simulink model "six_plus_six_AcmsteeringV09_main_2lfrf"  (R2014a)
settings: Solver=FixedStepDiscrete  StartTime=0.0  StopTime=10.0  FixedStep=0.0005  RelTol=1e-3
InitFcn:
  | Veh_Par_wxt
undefined symbols (not defined in the file or in its folder): acc_spdctl, ag_thr, B, bra_em, bra_pre_gz2, bra_pre_gz34, bra_pre_yd, brakepre_dem_data, brakeTrq_dem_data, bratrq_max, ecucoder_acal, eff_tran, ESP_switch, G, guzhang_lf, guzhang_lm, guzhang_lr, guzhang_rf, guzhang_rm, guzhang_rr, kd1, kd2, ki1, ki2, kp1, kp2, L, myFIS, premax, Radius, RC_switch, s_opt_yi, s_opt_zhuan, s_opt_zhuan_add, s_opt_zhuan_table, spd_map_mot, spd_spdctl, speed_thr_park, TCS_switch, tras_ratio, trq_map_mot, trqmax_yd, trqmax_zx, trqmaxneg, v_gain, v_table, v_thr_park, zhidong_bianmazhi, zhidong_down, zhidong_up, zhidong_youmen, zhuanxiang_bianmazhi, zhuanxiang_down, zhuanxiang_up, zhuanxiang_youmen
libraries: simulink x980, ec5744lib x59, fuzblock x2
(part 1 of 25)
settings Model: Creator=pc  LastModifiedBy=ZJK
settings OptimizationCC: InlineParams=on  InlineInvariantSignals=on  ExpressionFolding=off  RollThreshold=9  StateBitsets=on  DataBitsets=on  UseTempVars=on  ZeroExternalMemoryAtStartup=off  ZeroInternalMemoryAtStartup=off  EfficientFloat2IntCast=on  OptimizeModelRefInitCode=on  LifeSpan=1
settings DebuggingCC: InheritedTsInSrcMsg=none  MultiTaskDSMMsg=none
settings HardwareCC: ProdLargestAtomicInteger=Long  ProdLargestAtomicFloat=Double  ProdIntDivRoundTo=Zero  ProdEndianess=BigEndian  ProdHWDeviceType=Freescale MPC5500
settings RTWCC: SystemTargetFile=ec5744.tlc  MakeCommand=make_rtw optimized_fixed_point=1  GenerateMakefile=off  TemplateMakefile=ec5744_lcc.tmf  PostCodeGenCommand=ec5744_pst_s2(buildInfo)  Description=Target for EC5744  GenerateReport=on  ProcessScript=ec5744_make_rtw_hook  IncludeHyperlinkInReport=on  LaunchReport=on
settings CodeAppCC: IgnoreCustomStorageClasses=off
settings STFCustomTargetCC: ModelReferenceCompliant=off  ConcurrentExecutionCompliant=off  IncludeMdlTerminateFcn=off  GeneratePreprocessorConditionals=Use local settings  CombineOutputUpdateFcns=on  SuppressErrorStatus=on  ERTCustomFileBanners=on  SupportContinuousTime=off  SupportNonInlinedSFcns=off  MATLABClassNameForMDSCustomization=Simulink.SoftwareTarget.ERTCustomization  GRTInterface=off  SystemTargetFile=ec5744.tlc
settings ERTTargetCC: GenerateSampleERTMain=off  ModelReferenceCompliant=off  IncludeMdlTerminateFcn=off  SuppressErrorStatus=on  GenerateASAP2=on  ERTSrcFileBannerTemplate=ec5744_code_template.cgt  ERTHdrFileBannerTemplate=ec5744_code_template.cgt  ERTDataSrcFileTemplate=ec5744_code_template.cgt  ERTDataHdrFileTemplate=ec5744_code_template.cgt  ERTCustomFileTemplate=ec5744_file_process.tlc

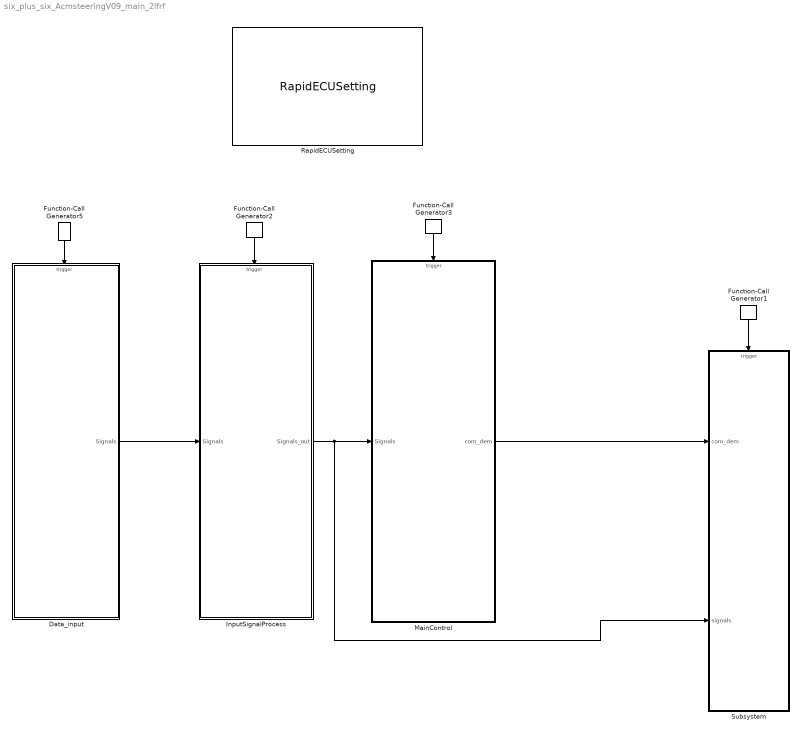
== system six_plus_six_AcmsteeringV09_main_2lfrf ==
  Data_input : Subsystem
  Function-Call Generator{1..3,5} (4 alike) : simulink/Ports & Subsystems/Function-Call Generator  sample_time=0.05  numberOfIterations=1
  InputSignalProcess : Subsystem  TreatAsAtomicUnit=on
  MainControl : Subsystem
  RapidECUSetting : ec5744lib/RapidECU_U3/RapidECUSetting
      link override CAN: apdf=4  bpdf=4  cpdf=4  acmt=Extended(29-bit ID)
      link override LIN: abrt=19200
  Subsystem : Subsystem
  wires:
  Function-Call Generator5/1 -> Data_input/Trigger
  Function-Call Generator1/1 -> Subsystem/Trigger
  Data_input/1(Signals) -> InputSignalProcess/1(Signals)
  Function-Call Generator2/1 -> InputSignalProcess/Trigger
  Function-Call Generator3/1 -> MainControl/Trigger
  InputSignalProcess/1(Signals_out) -> Subsystem/2("signals "), MainControl/1(Signals)
  MainControl/1(com_dem) -> Subsystem/1(com_dem)

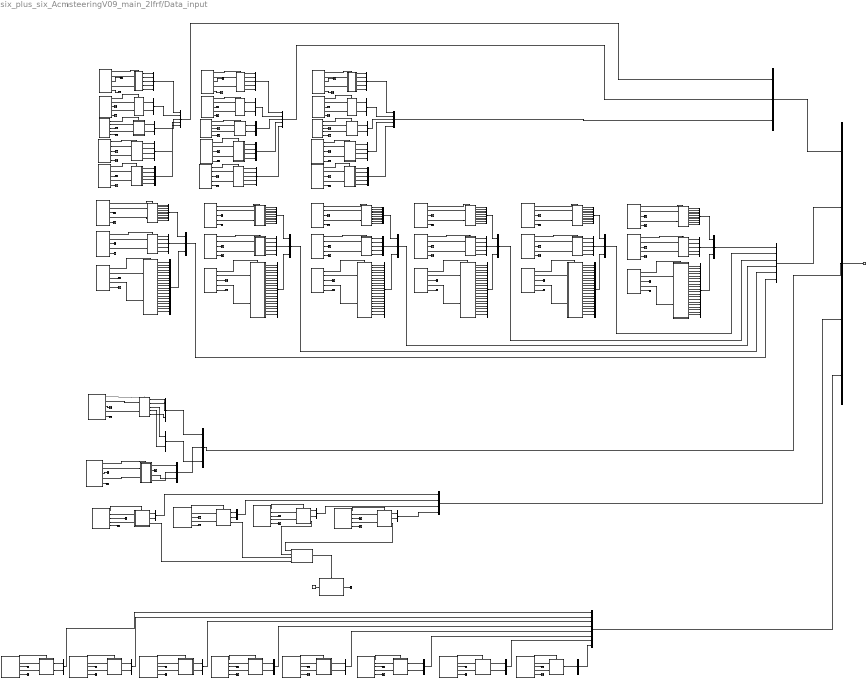
== system six_plus_six_AcmsteeringV09_main_2lfrf/Data_input ==
  note: 驱动电机1
  note: 电池管理系统主机1
  note: 电机报警信息
  note: 电机电气参数
  note: 电机状态信息
  note: 电池管理系统主机2
  note: 电池管理系统主机3
  note: 驱动电机2
  note: 电机报警信息
  note: 电机电气参数
  note: 电机状态信息
  note: 驱动电机3
  note: 电机报警信息
  note: 电机电气参数
  note: 电机状态信息
  note: 驱动电机4
  note: 电机报警信息
  note: 电机电气参数
  note: 电机状态信息
  note: 驱动电机5
  note: 电机报警信息
  note: 电机电气参数
  note: 电机状态信息
  note: 驱动电机6
  note: 电机报警信息
  note: 电机电气参数
  note: 电机状态信息
  note: 遥控器1
  note: SH/SE/ SD/SA/ 生命信号
  note: 遥控器2
  note: 左右摇杆
  note: motec转向电机1反馈报文
  note: motec转向电机2反馈报文
  note: motec转向电机3反馈报文
  note: motec制动电机反馈报文
  note: 进入OP模式，预设2s
  note: 组合惯导反馈报文1
  note: 组合惯导反馈报文2
  note: 组合惯导反馈报文3
  note: 组合惯导反馈报文4
  note: 组合惯导反馈报文5
  note: 组合惯导反馈报文6
  note: 组合惯导反馈报文7
  note: 组合惯导反馈报文8
  function : TriggerPort  TriggerType=function-call
  1 : Subsystem
  10 : Subsystem
  11 : Subsystem
  181 : Subsystem
  2 : Subsystem
  3 : Subsystem
  4 : Subsystem
  5 : Subsystem
  6 : Subsystem
  7 : Subsystem
  8 : Subsystem
  9 : Subsystem
  BMS1 : Subsystem
  BMS1-2 : Subsystem
  BMS1_1 : Subsystem
  BMS2 : Subsystem
  BMS2_1 : Subsystem
  BMS2_2 : Subsystem
  BMS3 : Subsystem
  BMS3_1 : Subsystem
  BMS3_2 : Subsystem
  BMS4 : Subsystem
  BMS4_1 : Subsystem
  BMS4_2 : Subsystem
  BMS5 : Subsystem
  BMS5_1 : Subsystem
  BMS5_2 : Subsystem
  Bus Creator{,22,25,28,31,34} (6 alike) : BusCreator  Inputs=10
  Bus Creator{1,3,7..9,13..15,19..20,23,26,29,32,35,44} (16 alike) : BusCreator  Inputs=5
  Bus Creator{4..5,10..11,16..17,47,49..52,57..63} (18 alike) : BusCreator  Inputs=2
  Bus Creator{6,12,18,53} (4 alike) : BusCreator
  Bus Creator{2,24,27,30,33,36} (6 alike) : BusCreator  Inputs=20
  Bus Creator{21,37..42,45..46,48} (10 alike) : BusCreator  Inputs=3
  Bus Creator43 : BusCreator  Inputs=6
  Bus Creator64 : BusCreator  Inputs=8
  Bus Creator65 : BusCreator  Inputs=1
  CANReceive : ec5744lib/RapidECU_U3/04CANCommunication/CANReceive  canmodule=0  canbuffer=23  canmessageid=hex2dec('CFA00EF')  canmessagetype=Extended(29-bit ID)  datalength=8  sampletime=-1
  CANReceive1 : ec5744lib/RapidECU_U3/04CANCommunication/CANReceive  canmodule=0  canbuffer=24  canmessageid=hex2dec('CFA01EF')  canmessagetype=Extended(29-bit ID)  datalength=8  sampletime=-1
  CANReceive10 : ec5744lib/RapidECU_U3/04CANCommunication/CANReceive  canmodule=1  canbuffer=7  canmessageid=hex2dec('42')  canmessagetype=Standard(11-bit ID)  datalength=8  sampletime=-1
  CANReceive11 : ec5744lib/RapidECU_U3/04CANCommunication/CANReceive  canmodule=1  canbuffer=16  canmessageid=hex2dec('52')  canmessagetype=Standard(11-bit ID)  datalength=8  sampletime=-1
  CANReceive12 : ec5744lib/RapidECU_U3/04CANCommunication/CANReceive  canmodule=1  canbuffer=17  canmessageid=hex2dec('62')  canmessagetype=Standard(11-bit ID)  datalength=8  sampletime=-1
  CANReceive13 : ec5744lib/RapidECU_U3/04CANCommunication/CANReceive  canmodule=1  canbuffer=18  canmessageid=hex2dec('23')  canmessagetype=Standard(11-bit ID)  datalength=8  sampletime=-1
  CANReceive14 : ec5744lib/RapidECU_U3/04CANCommunication/CANReceive  canmodule=1  canbuffer=19  canmessageid=hex2dec('33')  canmessagetype=Standard(11-bit ID)  datalength=8  sampletime=-1
  CANReceive15 : ec5744lib/RapidECU_U3/04CANCommunication/CANReceive  canmodule=1  canbuffer=20  canmessageid=hex2dec('43')  canmessagetype=Standard(11-bit ID)  datalength=8  sampletime=-1
  CANReceive16 : ec5744lib/RapidECU_U3/04CANCommunication/CANReceive  canmodule=1  canbuffer=21  canmessageid=hex2dec('53')  canmessagetype=Standard(11-bit ID)  datalength=8  sampletime=-1
  CANReceive17 : ec5744lib/RapidECU_U3/04CANCommunication/CANReceive  canmodule=1  canbuffer=22  canmessageid=hex2dec('63')  canmessagetype=Standard(11-bit ID)  datalength=8  sampletime=-1
  CANReceive18 : ec5744lib/RapidECU_U3/04CANCommunication/CANReceive  canmodule=0  canbuffer=26  canmessageid=hex2dec('CFA00F0')  canmessagetype=Extended(29-bit ID)  datalength=8  sampletime=-1
  CANReceive19 : ec5744lib/RapidECU_U3/04CANCommunication/CANReceive  canmodule=0  canbuffer=27  canmessageid=hex2dec('CFA01F0')  canmessagetype=Extended(29-bit ID)  datalength=8  sampletime=-1
  CANReceive2 : ec5744lib/RapidECU_U3/04CANCommunication/CANReceive  canmodule=0  canbuffer=25  canmessageid=hex2dec('18FA02EF')  canmessagetype=Extended(29-bit ID)  datalength=8  sampletime=-1
  CANReceive20 : ec5744lib/RapidECU_U3/04CANCommunication/CANReceive  canmodule=0  canbuffer=28  canmessageid=hex2dec('18FA02F0')  canmessagetype=Extended(29-bit ID)  datalength=8  sampletime=-1
  CANReceive21 : ec5744lib/RapidECU_U3/04CANCommunication/CANReceive  canmodule=0  canbuffer=29  canmessageid=hex2dec('CFA00F1')  canmessagetype=Extended(29-bit ID)  datalength=8  sampletime=-1
  CANReceive22 : ec5744lib/RapidECU_U3/04CANCommunication/CANReceive  canmodule=0  canbuffer=30  canmessageid=hex2dec('CFA01F1')  canmessagetype=Extended(29-bit ID)  datalength=8  sampletime=-1
  CANReceive23 : ec5744lib/RapidECU_U3/04CANCommunication/CANReceive  canmodule=0  canbuffer=31  canmessageid=hex2dec('18FA02F1')  canmessagetype=Extended(29-bit ID)  datalength=8  sampletime=-1
  CANReceive24 : ec5744lib/RapidECU_U3/04CANCommunication/CANReceive  canmodule=0  canbuffer=32  canmessageid=hex2dec('CFA00F2')  canmessagetype=Extended(29-bit ID)  datalength=8  sampletime=-1
  CANReceive25 : ec5744lib/RapidECU_U3/04CANCommunication/CANReceive  canmodule=0  canbuffer=33  canmessageid=hex2dec('CFA01F2')  canmessagetype=Extended(29-bit ID)  datalength=8  sampletime=-1
  CANReceive26 : ec5744lib/RapidECU_U3/04CANCommunication/CANReceive  canmodule=0  canbuffer=34  canmessageid=hex2dec('18FA02F2')  canmessagetype=Extended(29-bit ID)  datalength=8  sampletime=-1
  CANReceive27 : ec5744lib/RapidECU_U3/04CANCommunication/CANReceive  canmodule=0  canbuffer=35  canmessageid=hex2dec('CFA00F3')  canmessagetype=Extended(29-bit ID)  datalength=8  sampletime=-1
  CANReceive28 : ec5744lib/RapidECU_U3/04CANCommunication/CANReceive  canmodule=0  canbuffer=36  canmessageid=hex2dec('CFA01F3')  canmessagetype=Extended(29-bit ID)  datalength=8  sampletime=-1
  CANReceive29 : ec5744lib/RapidECU_U3/04CANCommunication/CANReceive  canmodule=0  canbuffer=37  canmessageid=hex2dec('18FA02F3')  canmessagetype=Extended(29-bit ID)  datalength=8  sampletime=-1
  CANReceive3 : ec5744lib/RapidECU_U3/04CANCommunication/CANReceive  canmodule=1  canbuffer=0  canmessageid=hex2dec('21')  canmessagetype=Standard(11-bit ID)  datalength=8  sampletime=-1
  CANReceive30 : ec5744lib/RapidECU_U3/04CANCommunication/CANReceive  canmodule=0  canbuffer=38  canmessageid=hex2dec('CFA00F4')  canmessagetype=Extended(29-bit ID)  datalength=8  sampletime=-1
  CANReceive31 : ec5744lib/RapidECU_U3/04CANCommunication/CANReceive  canmodule=0  canbuffer=39  canmessageid=hex2dec('CFA01F4')  canmessagetype=Extended(29-bit ID)  datalength=8  sampletime=-1
  CANReceive32 : ec5744lib/RapidECU_U3/04CANCommunication/CANReceive  canmodule=0  canbuffer=40  canmessageid=hex2dec('18FA02F4')  canmessagetype=Extended(29-bit ID)  datalength=8  sampletime=-1
  CANReceive33 : ec5744lib/RapidECU_U3/04CANCommunication/CANReceive  canmodule=1  canbuffer=42  canmessageid=hex2dec('11')  canmessagetype=Standard(11-bit ID)  datalength=8  sampletime=-1
  CANReceive34 : ec5744lib/RapidECU_U3/04CANCommunication/CANReceive  canmodule=1  canbuffer=41  canmessageid=hex2dec('12')  canmessagetype=Standard(11-bit ID)  datalength=8  sampletime=-1
  CANReceive35 : ec5744lib/RapidECU_U3/04CANCommunication/CANReceive  canmodule=1  canbuffer=43  canmessageid=hex2dec('0182')  canmessagetype=Standard(11-bit ID)  datalength=6  sampletime=-1
  CANReceive36 : ec5744lib/RapidECU_U3/04CANCommunication/CANReceive  canmodule=1  canbuffer=44  canmessageid=hex2dec('0183')  canmessagetype=Standard(11-bit ID)  datalength=6  sampletime=-1
  CANReceive37 : ec5744lib/RapidECU_U3/04CANCommunication/CANReceive  canmodule=1  canbuffer=45  canmessageid=hex2dec('0184')  canmessagetype=Standard(11-bit ID)  datalength=6  sampletime=-1
  CANReceive38 : ec5744lib/RapidECU_U3/04CANCommunication/CANReceive  canmodule=1  canbuffer=46  canmessageid=hex2dec('0181')  canmessagetype=Standard(11-bit ID)  datalength=6  sampletime=-1
  CANReceive4 : ec5744lib/RapidECU_U3/04CANCommunication/CANReceive  canmodule=1  canbuffer=1  canmessageid=hex2dec('31')  canmessagetype=Standard(11-bit ID)  datalength=8  sampletime=-1
  CANReceive40 : ec5744lib/RapidECU_U3/04CANCommunication/CANReceive  canmodule=1  canbuffer=47  canmessageid=hex2dec('100')  canmessagetype=Standard(11-bit ID)  datalength=8  sampletime=-1
  CANReceive42 : ec5744lib/RapidECU_U3/04CANCommunication/CANReceive  canmodule=1  canbuffer=48  canmessageid=hex2dec('101')  canmessagetype=Standard(11-bit ID)  datalength=8  sampletime=-1
  CANReceive43 : ec5744lib/RapidECU_U3/04CANCommunication/CANReceive  canmodule=1  canbuffer=49  canmessageid=hex2dec('102')  canmessagetype=Standard(11-bit ID)  datalength=8  sampletime=-1
  CANReceive44 : ec5744lib/RapidECU_U3/04CANCommunication/CANReceive  canmodule=1  canbuffer=50  canmessageid=hex2dec('103')  canmessagetype=Standard(11-bit ID)  datalength=8  sampletime=-1
  CANReceive45 : ec5744lib/RapidECU_U3/04CANCommunication/CANReceive  canmodule=1  canbuffer=51  canmessageid=hex2dec('104')  canmessagetype=Standard(11-bit ID)  datalength=8  sampletime=-1
  CANReceive46 : ec5744lib/RapidECU_U3/04CANCommunication/CANReceive  canmodule=1  canbuffer=52  canmessageid=hex2dec('105')  canmessagetype=Standard(11-bit ID)  datalength=8  sampletime=-1
  CANReceive47 : ec5744lib/RapidECU_U3/04CANCommunication/CANReceive  canmodule=1  canbuffer=53  canmessageid=hex2dec('106')  canmessagetype=Standard(11-bit ID)  datalength=8  sampletime=-1
  CANReceive48 : ec5744lib/RapidECU_U3/04CANCommunication/CANReceive  canmodule=1  canbuffer=54  canmessageid=hex2dec('107')  canmessagetype=Standard(11-bit ID)  datalength=8  sampletime=-1
  CANReceive5 : ec5744lib/RapidECU_U3/04CANCommunication/CANReceive  canmodule=1  canbuffer=2  canmessageid=hex2dec('41')  canmessagetype=Standard(11-bit ID)  datalength=8  sampletime=-1
  CANReceive6 : ec5744lib/RapidECU_U3/04CANCommunication/CANReceive  canmodule=1  canbuffer=3  canmessageid=hex2dec('51')  canmessagetype=Standard(11-bit ID)  datalength=8  sampletime=-1
  CANReceive7 : ec5744lib/RapidECU_U3/04CANCommunication/CANReceive  canmodule=1  canbuffer=4  canmessageid=hex2dec('61')  canmessagetype=Standard(11-bit ID)  datalength=8  sampletime=-1
  CANReceive8 : ec5744lib/RapidECU_U3/04CANCommunication/CANReceive  canmodule=1  canbuffer=5  canmessageid=hex2dec('22')  canmessagetype=Standard(11-bit ID)  datalength=8  sampletime=-1
  CANReceive9 : ec5744lib/RapidECU_U3/04CANCommunication/CANReceive  canmodule=1  canbuffer=6  canmessageid=hex2dec('32')  canmessagetype=Standard(11-bit ID)  datalength=8  sampletime=-1
  Constant1 : Constant  SampleTime=-1
  Enabled Subsystem : Subsystem  TreatAsAtomicUnit=on
  MATLAB Function : MATLAB Function  TreatAsAtomicUnit=on
  MCU0 : Subsystem
  MCU0_1 : Subsystem
  MCU0_2 : Subsystem
  MCU0_3 : Subsystem
  MCU0_4 : Subsystem
  MCU0_5 : Subsystem
  MCU1 : Subsystem
  MCU1_1 : Subsystem
  MCU1_2 : Subsystem
  MCU1_3 : Subsystem
  MCU1_4 : Subsystem
  MCU1_5 : Subsystem
  MCU2 : Subsystem
  MCU2_1 : Subsystem
  MCU2_2 : Subsystem
  MCU2_3 : Subsystem
  MCU2_4 : Subsystem
  MCU2_5 : Subsystem
  RemoteControl1 : Subsystem
  RemoteControl2 : Subsystem
  Terminator{,1..79,84..99} (96 alike) : Terminator
  Signals : Outport
  wires:
  CANReceive4/5 -> Terminator9/1
  CANReceive4/4 -> BMS2/2(In2)
  BMS5/1(BMS5_UpDownReuest) -> Bus Creator7/1  "BMS5_UpDownReuest"
  BMS5/5(BMS5_15s_InstanceDisPower) -> Bus Creator7/5  "BMS5_15s_InstanceDisPower"
  BMS5/4(BMS5_ContDischargePower) -> Bus Creator7/4  "BMS5_ContDischargePower"
  BMS1/4(BMS1_Sys_Status1) -> Bus Creator3/4  "BMS1_Sys_Status1"
  BMS1/5(BMS1_SOC) -> Bus Creator3/5  "BMS1_SOC"
  BMS5/2(BMS5_FeedbackPower) -> Bus Creator7/2  "BMS5_FeedbackPower"
  CANReceive3/2 -> BMS1/1(In1)
  BMS3/1(BMS3_LowTemperature) -> Bus Creator5/1  "BMS3_LowTemperature"
  CANReceive6/3 -> Terminator12/1
  CANReceive5/5 -> Terminator11/1
  CANReceive7/2 -> BMS5/1(In1)
  BMS4/4(BMS4_InputVolACC) -> Bus Creator6/4  "BMS4_InputVolACC"
  BMS4/1(BMS4_Sys_Status) -> Bus Creator6/1  "BMS4_Sys_Status"
  CANReceive4/3 -> Terminator8/1
  CANReceive4/2 -> BMS2/1(In1)
  BMS5/3(BMS5_FailureLevel) -> Bus Creator7/3  "BMS5_FailureLevel"
  CANReceive/4 -> MCU0/2(In2)
  CANReceive/3 -> Terminator/1
  CANReceive/5 -> Terminator1/1
  CANReceive/1 -> MCU0/Trigger
  MCU0/4(MCU_HighVol) -> Bus Creator/4  "MCU0_HighVol"
  MCU0/1(MCU0_TorqueMax) -> Bus Creator/1  "MCU0_TorqueMax"
  MCU0/5(MCU0_LiftCnt) -> Bus Creator/5  "MCU0_LiftCnt"
  MCU0/6(MCU0_torqueFdk) -> Bus Creator/6  "MCU0_TorqueFdk"
  MCU0/7(MCU0_SpeedFdk) -> Bus Creator/7  "MCU0_SpeedFdk"
  MCU0/2(MCU0_EmergShutDown) -> Bus Creator/2  "MCU0_EmergShutDown"
  MCU0/9(MCU0_ControlMode) -> Bus Creator/9  "MCU0_ControlMode"
  MCU0/10(MCU0_WorkStatus) -> Bus Creator/10  "MCU0_WorkStatus"
  CANReceive1/1 -> MCU1/Trigger
  CANReceive/2 -> MCU0/1(In1)
  MCU0/3(MCU_ShutDownAllow) -> Bus Creator/3  "MCU0_ShutDownAllow"
  MCU0/8(MCU0_GearStatus) -> Bus Creator/8  "MCU0_GearStatus"
  CANReceive2/3 -> Terminator4/1
  CANReceive1/4 -> MCU1/2(In2)
  CANReceive2/5 -> Terminator5/1
  MCU2/6(MCU2_luSensorFault) -> Bus Creator2/6  "MCU2_luSensorFault"
  MCU1/5(MCU_Udc) -> Bus Creator1/5  "MCU1_Udc"
  MCU2/4(MCU2_ActiveDischargingFault) -> Bus Creator2/4  "MCU2_ActiveDischargingFault"
  MCU2/10(MCU2_CanCommunicationFault) -> Bus Creator2/10  "MCU2_CanCommunicationFault"
  MCU2/15(MCU2_ControllerOverTemp) -> Bus Creator2/15  "MCU2_ControllerOverTemp"
  CANReceive1/3 -> Terminator2/1
  CANReceive1/2 -> MCU1/1(In1)
  MCU2/2(MCU2_UdcDetectionFault) -> Bus Creator2/2  "MCU2_UdcDetectionFault"
  MCU2/13(MCU2_IGBTFault) -> Bus Creator2/13  "MCU2_IGBTFault"
  MCU2/12(MCU2_DownratingFault) -> Bus Creator2/12  "MCU2_DownratingFault"
  CANReceive1/5 -> Terminator3/1
  MCU2/11(MCU2_MemoryFault) -> Bus Creator2/11  "MCU2_MemoryFault"
  MCU2/7(MCU2_lvSensorFault) -> Bus Creator2/7  "MCU2_lvSensorFault"
  MCU2/16(MCU2_MotorOverSpeed) -> Bus Creator2/16  "MCU2_MotorOverSpeed"
  MCU1/4(MCU1_idc) -> Bus Creator1/4  "MCU1_idc"
  MCU1/1(MCU1_ControlTemp) -> Bus Creator1/1  "MCU1_ControlTemp"
  CANReceive2/1 -> MCU2/Trigger
  MCU2/9(MCU2_Controllerload) -> Bus Creator2/9  "MCU2_Controllerload"
  MCU2/17(MCU2_RotaryInverterFault) -> Bus Creator2/17  "MCU2_RotaryInverterFault"
  MCU2/1(MCU2_MotorStallingFault) -> Bus Creator2/1  "MCU2_MotorStallingFault"
  CANReceive2/4 -> MCU2/2(In2)
  MCU2/5(MCU2_ldcSensorFault) -> Bus Creator2/5  "MCU2_ldcSensorFault"
  MCU2/8(MCU2_FaultLevel) -> Bus Creator2/8  "MCU2_FaultLevel"
  MCU2/14(MCU2_MotorOverTemp) -> Bus Creator2/14  "MCU2_MotorOverTemp"
  MCU1/2(MCU1_MotorTemp) -> Bus Creator1/2  "MCU1_MotorTemp"
  CANReceive2/2 -> MCU2/1(In1)
  MCU2/3(MCU2_TempSensorFault) -> Bus Creator2/3  "MCU2_TempSensorFault"
  MCU2/18(MCU2_UnderVoltage) -> Bus Creator2/18  "MCU2_UnderVoltage"
  MCU1/3(MCU_PowerFdk) -> Bus Creator1/3  "MCU1_PowerFdk"
  MCU2/20(MCU2_MotorOverLoad) -> Bus Creator2/20  "MCU2_MotorOverLoad"
  MCU2/19(MCU2_OverVoltage) -> Bus Creator2/19  "MCU2_OverVoltage"
  BMS3/2(BMS3_HighTemperature) -> Bus Creator5/2  "BMS3_HighTemperature"
  CANReceive3/5 -> Terminator6/1
  CANReceive3/3 -> Terminator7/1
  BMS1/2(BMS1_TotalCurrent) -> Bus Creator3/2  "BMS1_TotalCurrent"
  BMS1/3(BMS1_Sys_Status2) -> Bus Creator3/3  "BMS1_Sys_Status2"
  CANReceive3/1 -> BMS1/Trigger
  BMS1/1(BMS1_TotalVol) -> Bus Creator3/1  "BMS1_TotalVol"
  CANReceive3/4 -> BMS1/2(In2)
  CANReceive5/4 -> BMS3/2(In2)
  CANReceive5/2 -> BMS3/1(In1)
  CANReceive5/3 -> Terminator10/1
  BMS4/2(BMS4_InputVolKEYON) -> Bus Creator6/2  "BMS4_InputVolKEYON"
  CANReceive5/1 -> BMS3/Trigger
  BMS4/3(BMS4_InputVolCHG) -> Bus Creator6/3  "BMS4_InputVolCHG"
  CANReceive7/4 -> BMS5/2(In2)
  CANReceive7/5 -> Terminator15/1
  CANReceive7/3 -> Terminator14/1
  CANReceive6/4 -> BMS4/2(In2)
  CANReceive6/1 -> BMS4/Trigger
  CANReceive6/2 -> BMS4/1(In1)
  BMS2/1(BMS2_LowSingleVol) -> Bus Creator4/1  "BMS2_LowSingleVol"
  BMS2/2(BMS2_HighSingleVol) -> Bus Creator4/2  "BMS2_HighSingleVol"
  CANReceive7/1 -> BMS5/Trigger
  CANReceive6/5 -> Terminator13/1
  CANReceive4/1 -> BMS2/Trigger
  Bus Creator3/1 -> Bus Creator8/1  "BMS1"
  Bus Creator4/1 -> Bus Creator8/2  "BMS2"
  Bus Creator5/1 -> Bus Creator8/3  "BMS3"
  Bus Creator6/1 -> Bus Creator8/4  "BMS4"
  Bus Creator7/1 -> Bus Creator8/5  "BMS5"
  CANReceive9/5 -> Terminator25/1
  CANReceive9/4 -> BMS2_1/2(In2)
  BMS5_1/1(BMS5_UpDownReuest) -> Bus Creator13/1  "BMS5_1UpDownReuest"
  BMS5_1/5(BMS5_15s_InstanceDisPower) -> Bus Creator13/5  "BMS5_1_15s_InstanceDisPower"
  BMS5_1/4(BMS5_ContDischargePower) -> Bus Creator13/4  "BMS5_1ContDischargePower"
  BMS1_1/4(BMS1_Sys_Status1) -> Bus Creator9/4  "BMS1_1Sys_Status1"
  BMS1_1/5(BMS1_SOC) -> Bus Creator9/5  "BMS1_1SOC"
  BMS5_1/2(BMS5_FeedbackPower) -> Bus Creator13/2  "BMS5_1FeedbackPower"
  CANReceive8/2 -> BMS1_1/1(In1)
  BMS3_1/1(BMS3_LowTemperature) -> Bus Creator11/1  "BMS3_1LowTemperature"
  CANReceive11/3 -> Terminator18/1
  CANReceive10/5 -> Terminator17/1
  CANReceive12/2 -> BMS5_1/1(In1)
  BMS4_1/4(BMS4_InputVolACC) -> Bus Creator12/4  "BMS4_1InputVolACC"
  BMS4_1/1(BMS4_Sys_Status) -> Bus Creator12/1  "BMS4_1Sys_Status"
  CANReceive9/3 -> Terminator24/1
  CANReceive9/2 -> BMS2_1/1(In1)
  BMS5_1/3(BMS5_FailureLevel) -> Bus Creator13/3  "BMS5_1FailureLevel"
  BMS3_1/2(BMS3_HighTemperature) -> Bus Creator11/2  "BMS3_1HighTemperature"
  CANReceive8/5 -> Terminator22/1
  CANReceive8/3 -> Terminator23/1
  BMS1_1/2(BMS1_TotalCurrent) -> Bus Creator9/2  "BMS1_1TotalCurrent"
  BMS1_1/3(BMS1_Sys_Status2) -> Bus Creator9/3  "BMS1_1Sys_Status2"
  CANReceive8/1 -> BMS1_1/Trigger
  BMS1_1/1(BMS1_TotalVol) -> Bus Creator9/1  "BMS1_T1otalVol"
  CANReceive8/4 -> BMS1_1/2(In2)
  CANReceive10/4 -> BMS3_1/2(In2)
  CANReceive10/2 -> BMS3_1/1(In1)
  CANReceive10/3 -> Terminator16/1
  BMS4_1/2(BMS4_InputVolKEYON) -> Bus Creator12/2  "BMS4_1InputVolKEYON"
  CANReceive10/1 -> BMS3_1/Trigger
  BMS4_1/3(BMS4_InputVolCHG) -> Bus Creator12/3  "BMS4_1InputVolCHG"
  CANReceive12/4 -> BMS5_1/2(In2)
  CANReceive12/5 -> Terminator21/1
  CANReceive12/3 -> Terminator20/1
  CANReceive11/4 -> BMS4_1/2(In2)
  CANReceive11/1 -> BMS4_1/Trigger
  CANReceive11/2 -> BMS4_1/1(In1)
  BMS2_1/1(BMS2_LowSingleVol) -> Bus Creator10/1  "BMS2_1LowSingleVol"
  BMS2_1/2(BMS2_HighSingleVol) -> Bus Creator10/2  "BMS2_1HighSingleVol"
  CANReceive12/1 -> BMS5_1/Trigger
  CANReceive11/5 -> Terminator19/1
  CANReceive9/1 -> BMS2_1/Trigger
  CANReceive14/5 -> Terminator35/1
  CANReceive14/4 -> BMS2_2/2(In2)
  BMS5_2/1(BMS5_UpDownReuest) -> Bus Creator19/1  "BMS5_2UpDownReuest"
  BMS5_2/5(BMS5_15s_InstanceDisPower) -> Bus Creator19/5  "BMS5_2_15s_InstanceDisPower"
  BMS5_2/4(BMS5_ContDischargePower) -> Bus Creator19/4  "BMS5_2ContDischargePower"
  BMS1-2/4(BMS1_Sys_Status1) -> Bus Creator15/4  "BMS1_2Sys_Status1"
  BMS1-2/5(BMS1_SOC) -> Bus Creator15/5  "BMS1_2SOC"
  BMS5_2/2(BMS5_FeedbackPower) -> Bus Creator19/2  "BMS5_2FeedbackPower"
  CANReceive13/2 -> BMS1-2/1(In1)
  BMS3_2/1(BMS3_LowTemperature) -> Bus Creator17/1  "BMS3_2LowTemperature"
  CANReceive16/3 -> Terminator28/1
  CANReceive15/5 -> Terminator27/1
  CANReceive17/2 -> BMS5_2/1(In1)
  BMS4_2/4(BMS4_InputVolACC) -> Bus Creator18/4  "BMS4_2InputVolACC"
  BMS4_2/1(BMS4_Sys_Status) -> Bus Creator18/1  "BMS4_2Sys_Status"
  CANReceive14/3 -> Terminator34/1
  CANReceive14/2 -> BMS2_2/1(In1)
  BMS5_2/3(BMS5_FailureLevel) -> Bus Creator19/3  "BMS5_2FailureLevel"
  BMS3_2/2(BMS3_HighTemperature) -> Bus Creator17/2  "BMS3_2HighTemperature"
  CANReceive13/5 -> Terminator32/1
  CANReceive13/3 -> Terminator33/1
  BMS1-2/2(BMS1_TotalCurrent) -> Bus Creator15/2  "BMS1_2TotalCurrent"
  BMS1-2/3(BMS1_Sys_Status2) -> Bus Creator15/3  "BMS1_2Sys_Status2"
  CANReceive13/1 -> BMS1-2/Trigger
  BMS1-2/1(BMS1_TotalVol) -> Bus Creator15/1  "BMS1_2TotalVol"
  CANReceive13/4 -> BMS1-2/2(In2)
  CANReceive15/4 -> BMS3_2/2(In2)
  CANReceive15/2 -> BMS3_2/1(In1)
  CANReceive15/3 -> Terminator26/1
  BMS4_2/2(BMS4_InputVolKEYON) -> Bus Creator18/2  "BMS4_2InputVolKEYON"
  CANReceive15/1 -> BMS3_2/Trigger
  BMS4_2/3(BMS4_InputVolCHG) -> Bus Creator18/3  "BMS4_2InputVolCHG"
  CANReceive17/4 -> BMS5_2/2(In2)
  CANReceive17/5 -> Terminator31/1
  CANReceive17/3 -> Terminator30/1
  CANReceive16/4 -> BMS4_2/2(In2)
  CANReceive16/1 -> BMS4_2/Trigger
  CANReceive16/2 -> BMS4_2/1(In1)
  BMS2_2/1(BMS2_LowSingleVol) -> Bus Creator16/1  "BMS2_2LowSingleVol"
  BMS2_2/2(BMS2_HighSingleVol) -> Bus Creator16/2  "BMS2_2HighSingleVol"
  CANReceive17/1 -> BMS5_2/Trigger
  CANReceive16/5 -> Terminator29/1
  CANReceive14/1 -> BMS2_2/Trigger
  Bus Creator15/1 -> Bus Creator20/1  "BMS1_2"
  Bus Creator16/1 -> Bus Creator20/2  "BMS2_2"
  Bus Creator17/1 -> Bus Creator20/3  "BMS3_2"
  Bus Creator18/1 -> Bus Creator20/4  "BMS4_2"
  Bus Creator19/1 -> Bus Creator20/5  "BMS5_2"
  Bus Creator9/1 -> Bus Creator14/1  "BMS1_1"
  Bus Creator10/1 -> Bus Creator14/2  "BMS2_1"
  Bus Creator11/1 -> Bus Creator14/3  "BMS3_1"
  Bus Creator12/1 -> Bus Creator14/4  "BMS4_1"
  Bus Creator13/1 -> Bus Creator14/5  "BMS5_1"
  CANReceive18/4 -> MCU0_1/2(In2)
  CANReceive18/3 -> Terminator36/1
  CANReceive18/5 -> Terminator37/1
  CANReceive18/1 -> MCU0_1/Trigger
  MCU0_1/4(MCU_HighVol) -> Bus Creator22/4  "MCU0_1HighVol"
  MCU0_1/1(MCU0_TorqueMax) -> Bus Creator22/1  "MCU0_1TorqueMax"
  MCU0_1/5(MCU0_LiftCnt) -> Bus Creator22/5  "MCU0_1LiftCnt"
  MCU0_1/6(MCU0_torqueFdk) -> Bus Creator22/6  "MCU0_1TorqueFdk"
  MCU0_1/7(MCU0_SpeedFdk) -> Bus Creator22/7  "MCU0_1SpeedFdk"
  MCU0_1/2(MCU0_EmergShutDown) -> Bus Creator22/2  "MCU0_1EmergShutDown"
  MCU0_1/9(MCU0_ControlMode) -> Bus Creator22/9  "MCU0_1ControlMode"
  MCU0_1/10(MCU0_WorkStatus) -> Bus Creator22/10  "MCU0_1WorkStatus"
  CANReceive19/1 -> MCU1_1/Trigger
  CANReceive18/2 -> MCU0_1/1(In1)
  MCU0_1/3(MCU_ShutDownAllow) -> Bus Creator22/3  "MCU0_1ShutDownAllow"
  MCU0_1/8(MCU0_GearStatus) -> Bus Creator22/8  "MCU0_1GearStatus"
  CANReceive20/3 -> Terminator40/1
  CANReceive19/4 -> MCU1_1/2(In2)
  CANReceive20/5 -> Terminator41/1
  MCU2_1/6(MCU2_luSensorFault) -> Bus Creator24/6  "MCU2_1luSensorFault"
  MCU1_1/5(MCU_Udc) -> Bus Creator23/5  "MCU1_1Udc"
  MCU2_1/4(MCU2_ActiveDischargingFault) -> Bus Creator24/4  "MCU2_1ActiveDischargingFault"
  MCU2_1/10(MCU2_CanCommunicationFault) -> Bus Creator24/10  "MCU2_1CanCommunicationFault"
  MCU2_1/15(MCU2_ControllerOverTemp) -> Bus Creator24/15  "MCU2_1ControllerOverTemp"
  CANReceive19/3 -> Terminator38/1
  CANReceive19/2 -> MCU1_1/1(In1)
  MCU2_1/2(MCU2_UdcDetectionFault) -> Bus Creator24/2  "MCU2_1UdcDetectionFault"
  MCU2_1/13(MCU2_IGBTFault) -> Bus Creator24/13  "MCU2_1IGBTFault"
  MCU2_1/12(MCU2_DownratingFault) -> Bus Creator24/12  "MCU2_1DownratingFault"
  CANReceive19/5 -> Terminator39/1
  MCU2_1/11(MCU2_MemoryFault) -> Bus Creator24/11  "MCU2_1MemoryFault"
  MCU2_1/7(MCU2_lvSensorFault) -> Bus Creator24/7  "MCU2_1lvSensorFault"
  MCU2_1/16(MCU2_MotorOverSpeed) -> Bus Creator24/16  "MCU2_1MotorOverSpeed"
  MCU1_1/4(MCU1_idc) -> Bus Creator23/4  "MCU1_1idc"
  MCU1_1/1(MCU1_ControlTemp) -> Bus Creator23/1  "MCU1_1ControlTemp"
  CANReceive20/1 -> MCU2_1/Trigger
  MCU2_1/9(MCU2_Controllerload) -> Bus Creator24/9  "MCU2_1Controllerload"
  MCU2_1/17(MCU2_RotaryInverterFault) -> Bus Creator24/17  "MCU2_1RotaryInverterFault"
  MCU2_1/1(MCU2_MotorStallingFault) -> Bus Creator24/1  "MCU2_1MotorStallingFault"
  CANReceive20/4 -> MCU2_1/2(In2)
  MCU2_1/5(MCU2_ldcSensorFault) -> Bus Creator24/5  "MCU2_1ldcSensorFault"
  MCU2_1/8(MCU2_FaultLevel) -> Bus Creator24/8  "MCU2_1FaultLevel"
  MCU2_1/14(MCU2_MotorOverTemp) -> Bus Creator24/14  "MCU2_1MotorOverTemp"
  MCU1_1/2(MCU1_MotorTemp) -> Bus Creator23/2  "MCU1_1MotorTemp"
  CANReceive20/2 -> MCU2_1/1(In1)
  MCU2_1/3(MCU2_TempSensorFault) -> Bus Creator24/3  "MCU2_1TempSensorFault"
  MCU2_1/18(MCU2_UnderVoltage) -> Bus Creator24/18  "MCU2_1UnderVoltage"
  MCU1_1/3(MCU_PowerFdk) -> Bus Creator23/3  "MCU1_1PowerFdk"
  MCU2_1/20(MCU2_MotorOverLoad) -> Bus Creator24/20  "MCU2_1MotorOverLoad"
  MCU2_1/19(MCU2_OverVoltage) -> Bus Creator24/19  "MCU2_1OverVoltage"
  CANReceive21/4 -> MCU0_2/2(In2)
  CANReceive21/3 -> Terminator42/1
  CANReceive21/5 -> Terminator43/1
  CANReceive21/1 -> MCU0_2/Trigger
  MCU0_2/4(MCU_HighVol) -> Bus Creator25/4  "MCU0_2HighVol"
  MCU0_2/1(MCU0_TorqueMax) -> Bus Creator25/1  "MCU0_2TorqueMax"
  MCU0_2/5(MCU0_LiftCnt) -> Bus Creator25/5  "MCU0_2LiftCnt"
  MCU0_2/6(MCU0_torqueFdk) -> Bus Creator25/6  "MCU0_2TorqueFdk"
  MCU0_2/7(MCU0_SpeedFdk) -> Bus Creator25/7  "MCU0_2SpeedFdk"
  MCU0_2/2(MCU0_EmergShutDown) -> Bus Creator25/2  "MCU0_2EmergShutDown"
  MCU0_2/9(MCU0_ControlMode) -> Bus Creator25/9  "MCU0_2ControlMode"
  MCU0_2/10(MCU0_WorkStatus) -> Bus Creator25/10  "MCU0_2WorkStatus"
  CANReceive22/1 -> MCU1_2/Trigger
  CANReceive21/2 -> MCU0_2/1(In1)
  MCU0_2/3(MCU_ShutDownAllow) -> Bus Creator25/3  "MCU0_2ShutDownAllow"
  MCU0_2/8(MCU0_GearStatus) -> Bus Creator25/8  "MCU0_2GearStatus"
  CANReceive23/3 -> Terminator46/1
  CANReceive22/4 -> MCU1_2/2(In2)
  CANReceive23/5 -> Terminator47/1
  MCU2_2/6(MCU2_luSensorFault) -> Bus Creator27/6  "MCU2_2luSensorFault"
  MCU1_2/5(MCU_Udc) -> Bus Creator26/5  "MCU1_2Udc"
  MCU2_2/4(MCU2_ActiveDischargingFault) -> Bus Creator27/4  "MCU2_2ActiveDischargingFault"
  MCU2_2/10(MCU2_CanCommunicationFault) -> Bus Creator27/10  "MCU2_2CanCommunicationFault"
  MCU2_2/15(MCU2_ControllerOverTemp) -> Bus Creator27/15  "MCU2_2ControllerOverTemp"
  CANReceive22/3 -> Terminator44/1
  CANReceive22/2 -> MCU1_2/1(In1)
  MCU2_2/2(MCU2_UdcDetectionFault) -> Bus Creator27/2  "MCU2_2UdcDetectionFault"
  MCU2_2/13(MCU2_IGBTFault) -> Bus Creator27/13  "MCU2_2IGBTFault"
  MCU2_2/12(MCU2_DownratingFault) -> Bus Creator27/12  "MCU2_2DownratingFault"
  CANReceive22/5 -> Terminator45/1
  MCU2_2/11(MCU2_MemoryFault) -> Bus Creator27/11  "MCU2_2MemoryFault"
  MCU2_2/7(MCU2_lvSensorFault) -> Bus Creator27/7  "MCU2_2lvSensorFault"
  MCU2_2/16(MCU2_MotorOverSpeed) -> Bus Creator27/16  "MCU2_2MotorOverSpeed"
  MCU1_2/4(MCU1_idc) -> Bus Creator26/4  "MCU1_2idc"
  MCU1_2/1(MCU1_ControlTemp) -> Bus Creator26/1  "MCU1_2ControlTemp"
  CANReceive23/1 -> MCU2_2/Trigger
  MCU2_2/9(MCU2_Controllerload) -> Bus Creator27/9  "MCU2_2Controllerload"
  MCU2_2/17(MCU2_RotaryInverterFault) -> Bus Creator27/17  "MCU2_2RotaryInverterFault"
  MCU2_2/1(MCU2_MotorStallingFault) -> Bus Creator27/1  "MCU2_2MotorStallingFault"
  CANReceive23/4 -> MCU2_2/2(In2)
  MCU2_2/5(MCU2_ldcSensorFault) -> Bus Creator27/5  "MCU2_2ldcSensorFault"
  MCU2_2/8(MCU2_FaultLevel) -> Bus Creator27/8  "MCU2_2FaultLevel"
  MCU2_2/14(MCU2_MotorOverTemp) -> Bus Creator27/14  "MCU2_2MotorOverTemp"
  MCU1_2/2(MCU1_MotorTemp) -> Bus Creator26/2  "MCU1_2MotorTemp"
  CANReceive23/2 -> MCU2_2/1(In1)
  MCU2_2/3(MCU2_TempSensorFault) -> Bus Creator27/3  "MCU2_2TempSensorFault"
  MCU2_2/18(MCU2_UnderVoltage) -> Bus Creator27/18  "MCU2_2UnderVoltage"
  MCU1_2/3(MCU_PowerFdk) -> Bus Creator26/3  "MCU1_2PowerFdk"
  MCU2_2/20(MCU2_MotorOverLoad) -> Bus Creator27/20  "MCU2_2MotorOverLoad"
  MCU2_2/19(MCU2_OverVoltage) -> Bus Creator27/19  "MCU2_OverVoltage"
  CANReceive24/4 -> MCU0_3/2(In2)
  CANReceive24/3 -> Terminator48/1
  CANReceive24/5 -> Terminator49/1
  CANReceive24/1 -> MCU0_3/Trigger
  MCU0_3/4(MCU_HighVol) -> Bus Creator28/4  "MCU0_3HighVol"
  MCU0_3/1(MCU0_TorqueMax) -> Bus Creator28/1  "MCU0_3TorqueMax"
  MCU0_3/5(MCU0_LiftCnt) -> Bus Creator28/5  "MCU0_3LiftCnt"
  MCU0_3/6(MCU0_torqueFdk) -> Bus Creator28/6  "MCU0_3TorqueFdk"
  MCU0_3/7(MCU0_SpeedFdk) -> Bus Creator28/7  "MCU0_3SpeedFdk"
  MCU0_3/2(MCU0_EmergShutDown) -> Bus Creator28/2  "MCU0_3EmergShutDown"
  MCU0_3/9(MCU0_ControlMode) -> Bus Creator28/9  "MCU0_3ControlMode"
  MCU0_3/10(MCU0_WorkStatus) -> Bus Creator28/10  "MCU0_3WorkStatus"
  CANReceive25/1 -> MCU1_3/Trigger
  CANReceive24/2 -> MCU0_3/1(In1)
  MCU0_3/3(MCU_ShutDownAllow) -> Bus Creator28/3  "MCU0_3ShutDownAllow"
  MCU0_3/8(MCU0_GearStatus) -> Bus Creator28/8  "MCU0_3GearStatus"
  CANReceive26/3 -> Terminator52/1
  CANReceive25/4 -> MCU1_3/2(In2)
  CANReceive26/5 -> Terminator53/1
  MCU2_3/6(MCU2_luSensorFault) -> Bus Creator30/6  "MCU2_3luSensorFault"
  MCU1_3/5(MCU_Udc) -> Bus Creator29/5  "MCU1_3Udc"
  MCU2_3/4(MCU2_ActiveDischargingFault) -> Bus Creator30/4  "MCU2_3ActiveDischargingFault"
  MCU2_3/10(MCU2_CanCommunicationFault) -> Bus Creator30/10  "MCU2_3CanCommunicationFault"
  MCU2_3/15(MCU2_ControllerOverTemp) -> Bus Creator30/15  "MCU2_3ControllerOverTemp"
  CANReceive25/3 -> Terminator50/1
  CANReceive25/2 -> MCU1_3/1(In1)
  MCU2_3/2(MCU2_UdcDetectionFault) -> Bus Creator30/2  "MCU2_3UdcDetectionFault"
  MCU2_3/13(MCU2_IGBTFault) -> Bus Creator30/13  "MCU2_3IGBTFault"
  MCU2_3/12(MCU2_DownratingFault) -> Bus Creator30/12  "MCU2_3DownratingFault"
  CANReceive25/5 -> Terminator51/1
  MCU2_3/11(MCU2_MemoryFault) -> Bus Creator30/11  "MCU2_3MemoryFault"
  MCU2_3/7(MCU2_lvSensorFault) -> Bus Creator30/7  "MCU2_3lvSensorFault"
  MCU2_3/16(MCU2_MotorOverSpeed) -> Bus Creator30/16  "MCU2_3MotorOverSpeed"
  MCU1_3/4(MCU1_idc) -> Bus Creator29/4  "MCU1_3idc"
  MCU1_3/1(MCU1_ControlTemp) -> Bus Creator29/1  "MCU1_3ControlTemp"
  CANReceive26/1 -> MCU2_3/Trigger
  MCU2_3/9(MCU2_Controllerload) -> Bus Creator30/9  "MCU2_3Controllerload"
  MCU2_3/17(MCU2_RotaryInverterFault) -> Bus Creator30/17  "MCU2_3RotaryInverterFault"
  MCU2_3/1(MCU2_MotorStallingFault) -> Bus Creator30/1  "MCU2_3MotorStallingFault"
  CANReceive26/4 -> MCU2_3/2(In2)
  MCU2_3/5(MCU2_ldcSensorFault) -> Bus Creator30/5  "MCU2_3ldcSensorFault"
  MCU2_3/8(MCU2_FaultLevel) -> Bus Creator30/8  "MCU2_3FaultLevel"
  MCU2_3/14(MCU2_MotorOverTemp) -> Bus Creator30/14  "MCU2_3MotorOverTemp"
  MCU1_3/2(MCU1_MotorTemp) -> Bus Creator29/2  "MCU1_3MotorTemp"
  CANReceive26/2 -> MCU2_3/1(In1)
  MCU2_3/3(MCU2_TempSensorFault) -> Bus Creator30/3  "MCU2_3TempSensorFault"
  MCU2_3/18(MCU2_UnderVoltage) -> Bus Creator30/18  "MCU2_3UnderVoltage"
  MCU1_3/3(MCU_PowerFdk) -> Bus Creator29/3  "MCU1_3PowerFdk"
  MCU2_3/20(MCU2_MotorOverLoad) -> Bus Creator30/20  "MCU2_3MotorOverLoad"
  MCU2_3/19(MCU2_OverVoltage) -> Bus Creator30/19  "MCU2_3OverVoltage"
  CANReceive27/4 -> MCU0_4/2(In2)
  CANReceive27/3 -> Terminator54/1
  CANReceive27/5 -> Terminator55/1
  CANReceive27/1 -> MCU0_4/Trigger
  MCU0_4/4(MCU_HighVol) -> Bus Creator31/4  "MCU0_4HighVol"
  MCU0_4/1(MCU0_TorqueMax) -> Bus Creator31/1  "MCU0_4TorqueMax"
  MCU0_4/5(MCU0_LiftCnt) -> Bus Creator31/5  "MCU0_4LiftCnt"
  MCU0_4/6(MCU0_torqueFdk) -> Bus Creator31/6  "MCU0_4TorqueFdk"
  MCU0_4/7(MCU0_SpeedFdk) -> Bus Creator31/7  "MCU0_4SpeedFdk"
  MCU0_4/2(MCU0_EmergShutDown) -> Bus Creator31/2  "MCU0_4EmergShutDown"
  MCU0_4/9(MCU0_ControlMode) -> Bus Creator31/9  "MCU0_4ControlMode"
  MCU0_4/10(MCU0_WorkStatus) -> Bus Creator31/10  "MCU0_4WorkStatus"
  CANReceive28/1 -> MCU1_4/Trigger
  CANReceive27/2 -> MCU0_4/1(In1)
  MCU0_4/3(MCU_ShutDownAllow) -> Bus Creator31/3  "MCU0_4ShutDownAllow"
  MCU0_4/8(MCU0_GearStatus) -> Bus Creator31/8  "MCU0_4GearStatus"
  CANReceive29/3 -> Terminator58/1
  CANReceive28/4 -> MCU1_4/2(In2)
  CANReceive29/5 -> Terminator59/1
  MCU2_4/6(MCU2_luSensorFault) -> Bus Creator33/6  "MCU2_4luSensorFault"
  MCU1_4/5(MCU_Udc) -> Bus Creator32/5  "MCU1_4Udc"
  MCU2_4/4(MCU2_ActiveDischargingFault) -> Bus Creator33/4  "MCU2_4ActiveDischargingFault"
  MCU2_4/10(MCU2_CanCommunicationFault) -> Bus Creator33/10  "MCU2_4CanCommunicationFault"
  MCU2_4/15(MCU2_ControllerOverTemp) -> Bus Creator33/15  "MCU2_4ControllerOverTemp"
  CANReceive28/3 -> Terminator56/1
  CANReceive28/2 -> MCU1_4/1(In1)
  MCU2_4/2(MCU2_UdcDetectionFault) -> Bus Creator33/2  "MCU2_4UdcDetectionFault"
  MCU2_4/13(MCU2_IGBTFault) -> Bus Creator33/13  "MCU2_4IGBTFault"
  MCU2_4/12(MCU2_DownratingFault) -> Bus Creator33/12  "MCU2_4DownratingFault"
  CANReceive28/5 -> Terminator57/1
  MCU2_4/11(MCU2_MemoryFault) -> Bus Creator33/11  "MCU2_4MemoryFault"
  MCU2_4/7(MCU2_lvSensorFault) -> Bus Creator33/7  "MCU2_4lvSensorFault"
  MCU2_4/16(MCU2_MotorOverSpeed) -> Bus Creator33/16  "MCU2_4MotorOverSpeed"
  MCU1_4/4(MCU1_idc) -> Bus Creator32/4  "MCU1_4idc"
  MCU1_4/1(MCU1_ControlTemp) -> Bus Creator32/1  "MCU1_4ControlTemp"
  CANReceive29/1 -> MCU2_4/Trigger
  MCU2_4/9(MCU2_Controllerload) -> Bus Creator33/9  "MCU2_4Controllerload"
  MCU2_4/17(MCU2_RotaryInverterFault) -> Bus Creator33/17  "MCU2_4RotaryInverterFault"
  MCU2_4/1(MCU2_MotorStallingFault) -> Bus Creator33/1  "MCU2_4MotorStallingFault"
  CANReceive29/4 -> MCU2_4/2(In2)
  MCU2_4/5(MCU2_ldcSensorFault) -> Bus Creator33/5  "MCU2_4ldcSensorFault"
  MCU2_4/8(MCU2_FaultLevel) -> Bus Creator33/8  "MCU2_4FaultLevel"
  MCU2_4/14(MCU2_MotorOverTemp) -> Bus Creator33/14  "MCU2_4MotorOverTemp"
  MCU1_4/2(MCU1_MotorTemp) -> Bus Creator32/2  "MCU1_4MotorTemp"
  CANReceive29/2 -> MCU2_4/1(In1)
  MCU2_4/3(MCU2_TempSensorFault) -> Bus Creator33/3  "MCU2_4TempSensorFault"
  MCU2_4/18(MCU2_UnderVoltage) -> Bus Creator33/18  "MCU2_4UnderVoltage"
  MCU1_4/3(MCU_PowerFdk) -> Bus Creator32/3  "MCU1_4PowerFdk"
  MCU2_4/20(MCU2_MotorOverLoad) -> Bus Creator33/20  "MCU2_4MotorOverLoad"
  MCU2_4/19(MCU2_OverVoltage) -> Bus Creator33/19  "MCU2_4OverVoltage"
  CANReceive30/4 -> MCU0_5/2(In2)
  CANReceive30/3 -> Terminator60/1
  CANReceive30/5 -> Terminator61/1
  CANReceive30/1 -> MCU0_5/Trigger
  MCU0_5/4(MCU_HighVol) -> Bus Creator34/4  "MCU0_5HighVol"
  MCU0_5/1(MCU0_TorqueMax) -> Bus Creator34/1  "MCU0_5TorqueMax"
  MCU0_5/5(MCU0_LiftCnt) -> Bus Creator34/5  "MCU0_5LiftCnt"
  MCU0_5/6(MCU0_torqueFdk) -> Bus Creator34/6  "MCU0_5TorqueFdk"
  MCU0_5/7(MCU0_SpeedFdk) -> Bus Creator34/7  "MCU0_5SpeedFdk"
  MCU0_5/2(MCU0_EmergShutDown) -> Bus Creator34/2  "MCU0_5EmergShutDown"
  MCU0_5/9(MCU0_ControlMode) -> Bus Creator34/9  "MCU0_5ControlMode"
  MCU0_5/10(MCU0_WorkStatus) -> Bus Creator34/10  "MCU0_5WorkStatus"
  CANReceive31/1 -> MCU1_5/Trigger
  CANReceive30/2 -> MCU0_5/1(In1)
  MCU0_5/3(MCU_ShutDownAllow) -> Bus Creator34/3  "MCU0_5ShutDownAllow"
  MCU0_5/8(MCU0_GearStatus) -> Bus Creator34/8  "MCU0_5GearStatus"
  CANReceive32/3 -> Terminator64/1
  CANReceive31/4 -> MCU1_5/2(In2)
  CANReceive32/5 -> Terminator65/1
  MCU2_5/6(MCU2_luSensorFault) -> Bus Creator36/6  "MCU2_5luSensorFault"
  MCU1_5/5(MCU_Udc) -> Bus Creator35/5  "MCU1_5Udc"
  MCU2_5/4(MCU2_ActiveDischargingFault) -> Bus Creator36/4  "MCU2_5ActiveDischargingFault"
  MCU2_5/10(MCU2_CanCommunicationFault) -> Bus Creator36/10  "MCU2_5CanCommunicationFault"
  MCU2_5/15(MCU2_ControllerOverTemp) -> Bus Creator36/15  "MCU2_5ControllerOverTemp"
  CANReceive31/3 -> Terminator62/1
  CANReceive31/2 -> MCU1_5/1(In1)
  MCU2_5/2(MCU2_UdcDetectionFault) -> Bus Creator36/2  "MCU2_5UdcDetectionFault"
  MCU2_5/13(MCU2_IGBTFault) -> Bus Creator36/13  "MCU2_5IGBTFault"
  MCU2_5/12(MCU2_DownratingFault) -> Bus Creator36/12  "MCU2_5DownratingFault"
  CANReceive31/5 -> Terminator63/1
  MCU2_5/11(MCU2_MemoryFault) -> Bus Creator36/11  "MCU2_5MemoryFault"
  MCU2_5/7(MCU2_lvSensorFault) -> Bus Creator36/7  "MCU2_5lvSensorFault"
  MCU2_5/16(MCU2_MotorOverSpeed) -> Bus Creator36/16  "MCU2_5MotorOverSpeed"
  MCU1_5/4(MCU1_idc) -> Bus Creator35/4  "MCU1_5idc"
  MCU1_5/1(MCU1_ControlTemp) -> Bus Creator35/1  "MCU1_5ControlTemp"
  CANReceive32/1 -> MCU2_5/Trigger
  MCU2_5/9(MCU2_Controllerload) -> Bus Creator36/9  "MCU2_5Controllerload"
  MCU2_5/17(MCU2_RotaryInverterFault) -> Bus Creator36/17  "MCU2_5RotaryInverterFault"
  MCU2_5/1(MCU2_MotorStallingFault) -> Bus Creator36/1  "MCU2_5MotorStallingFault"
  CANReceive32/4 -> MCU2_5/2(In2)
  MCU2_5/5(MCU2_ldcSensorFault) -> Bus Creator36/5  "MCU2_5ldcSensorFault"
  MCU2_5/8(MCU2_FaultLevel) -> Bus Creator36/8  "MCU2_5FaultLevel"
  MCU2_5/14(MCU2_MotorOverTemp) -> Bus Creator36/14  "MCU2_5MotorOverTemp"
  MCU1_5/2(MCU1_MotorTemp) -> Bus Creator35/2  "MCU1_5MotorTemp"
  CANReceive32/2 -> MCU2_5/1(In1)
  MCU2_5/3(MCU2_TempSensorFault) -> Bus Creator36/3  "MCU2_5TempSensorFault"
  MCU2_5/18(MCU2_UnderVoltage) -> Bus Creator36/18  "MCU2_5UnderVoltage"
  MCU1_5/3(MCU_PowerFdk) -> Bus Creator35/3  "MCU1_5PowerFdk"
  MCU2_5/20(MCU2_MotorOverLoad) -> Bus Creator36/20  "MCU2_5MotorOverLoad"
  MCU2_5/19(MCU2_OverVoltage) -> Bus Creator36/19  "MCU2_5OverVoltage"
  Bus Creator/1 -> Bus Creator37/1  "MCU0"
  Bus Creator1/1 -> Bus Creator37/2  "MCU1"
  Bus Creator2/1 -> Bus Creator37/3  "MCU2"
  Bus Creator23/1 -> Bus Creator38/2  "MCU1_1"
  Bus Creator24/1 -> Bus Creator38/3  "MCU2_1"
  Bus Creator22/1 -> Bus Creator38/1  "MCU0_1"
  Bus Creator26/1 -> Bus Creator39/2  "MCU1_2"
  Bus Creator25/1 -> Bus Creator39/1  "MCU0_2"
  Bus Creator27/1 -> Bus Creator39/3  "MCU2-2"
  Bus Creator29/1 -> Bus Creator40/2  "MCU1_3"
  Bus Creator30/1 -> Bus Creator40/3  "MCU2_3"
  Bus Creator28/1 -> Bus Creator40/1  "MCU0_3"
  Bus Creator32/1 -> Bus Creator41/2  "MCU1_4"
  Bus Creator31/1 -> Bus Creator41/1  "MCU0_4"
  Bus Creator33/1 -> Bus Creator41/3  "MCU2_4"
  Bus Creator35/1 -> Bus Creator42/2  "MCU1_5"
  Bus Creator34/1 -> Bus Creator42/1  "MCU0_5"
  Bus Creator36/1 -> Bus Creator42/3  "MCU2_5"
  Bus Creator37/1 -> Bus Creator43/6  "MOTOR1"
  Bus Creator38/1 -> Bus Creator43/5  "MOTOR2"
  Bus Creator39/1 -> Bus Creator43/4  "MOTOR3"
  Bus Creator40/1 -> Bus Creator43/3  "MOTOR4"
  Bus Creator41/1 -> Bus Creator43/2  "MOTOR5"
  Bus Creator42/1 -> Bus Creator43/1  "MOTOR6"
  Bus Creator43/1 -> Bus Creator44/2  "MOTOR"
  Bus Creator21/1 -> Bus Creator44/1  "CCM"
  Bus Creator44/1 -> Signals/1
  CANReceive33/4 -> RemoteControl1/2(In2)
  CANReceive33/3 -> Terminator66/1
  CANReceive33/5 -> Terminator67/1
  CANReceive33/1 -> RemoteControl1/Trigger
  CANReceive33/2 -> RemoteControl1/1(In1)
  Bus Creator45/1 -> Bus Creator48/1  "RemoteControl1"
  RemoteControl1/1(SH) -> Bus Creator45/1  "SH"
  RemoteControl1/2(SE) -> Bus Creator45/2  "SE"
  RemoteControl1/5(LIFEspan) -> Bus Creator45/3  "LifeSpan"
  CANReceive34/4 -> RemoteControl2/2(In2)
  CANReceive34/3 -> Terminator68/1
  CANReceive34/5 -> Terminator69/1
  CANReceive34/1 -> RemoteControl2/Trigger
  CANReceive34/2 -> RemoteControl2/1(In1)
  Bus Creator46/1 -> Bus Creator48/2  "RemoteControl2"
  RemoteControl2/4(Leftstick_leftright) -> Bus Creator46/2  "LeftJoystick_LeftRight"
  RemoteControl2/3(Leftstick_updown) -> Bus Creator46/3  "LeftJoystick_UpDown"
  Bus Creator47/1 -> Bus Creator48/3  "RemoteControl3"
  RemoteControl1/3(SD) -> Bus Creator47/1  "SD"
  RemoteControl1/4(SA) -> Bus Creator47/2  "SA"
  Bus Creator48/1 -> Bus Creator44/3  "RemoteControl"
  Bus Creator8/1 -> Bus Creator21/1  "CCM1"
  Bus Creator14/1 -> Bus Creator21/2  "CCM2"
  Bus Creator20/1 -> Bus Creator21/3  "CCM3"
  RemoteControl2/2(Rightstick_leftright) -> Terminator70/1
  CANReceive35/3 -> Terminator71/1
  CANReceive35/1 -> 181/Trigger
  CANReceive35/2 -> 181/1(In1)
  CANReceive35/5 -> Terminator72/1
  CANReceive35/4 -> 181/2(In2)
  181/1(motec_spd_1) -> Bus Creator49/1  "motec_spd_1"
  181/2(motec_current_1) -> Bus Creator49/2  "motec_current_1"
  CANReceive36/3 -> Terminator73/1
  CANReceive36/1 -> 1/Trigger
  CANReceive36/2 -> 1/1(In1)
  CANReceive36/5 -> Terminator74/1
  CANReceive36/4 -> 1/2(In2)
  1/1(motec_spd_2) -> Bus Creator50/1  "motec_spd_2"
  1/2(motec_current_2) -> Bus Creator50/2  "motec_current_2"
  CANReceive37/3 -> Terminator75/1
  CANReceive37/1 -> 3/Trigger
  CANReceive37/2 -> 3/1(In1)
  CANReceive37/5 -> Terminator76/1
  CANReceive37/4 -> 3/2(In2)
  3/1(motec_spd_3) -> Bus Creator51/1  "motec_spd_3"
  3/2(motec_current_3) -> Bus Creator51/2  "motec_current_3"
  CANReceive38/3 -> Terminator77/1
  CANReceive38/1 -> 2/Trigger
  CANReceive38/2 -> 2/1(In1)
  CANReceive38/5 -> Terminator78/1
  CANReceive38/4 -> 2/2(In2)
  2/1(motec_spd_4) -> Bus Creator52/1  "motec_spd_4"
  2/2(motec_current_4) -> Bus Creator52/2  "motec_current_4"
  Bus Creator49/1 -> Bus Creator53/1  "motec1"
  Bus Creator50/1 -> Bus Creator53/2  "motec2"
  Bus Creator51/1 -> Bus Creator53/3  "motec3"
  Bus Creator52/1 -> Bus Creator53/4  "motec4"
  Bus Creator53/1 -> Bus Creator44/4  "motec"
  Constant1/1 -> Enabled Subsystem/1(In1)
  MATLAB Function/1(y) -> Enabled Subsystem/Enable
  Enabled Subsystem/1(Out1) -> Terminator79/1
  181/3(enable_count1) -> MATLAB Function/4(u4)
  1/3(enable_count) -> MATLAB Function/3(u3)
  2/3(enable_count) -> MATLAB Function/1(u1)
  3/3(enable_count3) -> MATLAB Function/2(u2)
  RemoteControl2/1(Rightstick_updown) -> Bus Creator46/1  "RirhtJoystick_UpDown"
  CANReceive40/3 -> Terminator84/1
  CANReceive40/1 -> 4/Trigger
  CANReceive40/2 -> 4/1(In1)
  CANReceive40/5 -> Terminator85/1
  CANReceive40/4 -> 4/2(In2)
  CANReceive42/3 -> Terminator86/1
  CANReceive42/1 -> 5/Trigger
  CANReceive42/2 -> 5/1(In1)
  CANReceive42/5 -> Terminator87/1
  CANReceive42/4 -> 5/2(In2)
  CANReceive43/3 -> Terminator88/1
  CANReceive43/1 -> 6/Trigger
  CANReceive43/2 -> 6/1(In1)
  CANReceive43/5 -> Terminator89/1
  CANReceive43/4 -> 6/2(In2)
  CANReceive44/3 -> Terminator90/1
  CANReceive44/1 -> 7/Trigger
  CANReceive44/2 -> 7/1(In1)
  CANReceive44/5 -> Terminator91/1
  CANReceive44/4 -> 7/2(In2)
  CANReceive45/3 -> Terminator92/1
  CANReceive45/1 -> 8/Trigger
  CANReceive45/2 -> 8/1(In1)
  CANReceive45/5 -> Terminator93/1
  CANReceive45/4 -> 8/2(In2)
  CANReceive46/3 -> Terminator94/1
  CANReceive46/1 -> 9/Trigger
  CANReceive46/2 -> 9/1(In1)
  CANReceive46/5 -> Terminator95/1
  CANReceive46/4 -> 9/2(In2)
  CANReceive47/3 -> Terminator96/1
  CANReceive47/1 -> 10/Trigger
  CANReceive47/2 -> 10/1(In1)
  CANReceive47/5 -> Terminator97/1
  CANReceive47/4 -> 10/2(In2)
  CANReceive48/3 -> Terminator98/1
  CANReceive48/1 -> 11/Trigger
  CANReceive48/2 -> 11/1(In1)
  CANReceive48/5 -> Terminator99/1
  CANReceive48/4 -> 11/2(In2)
  4/1(Xangularrate_Out) -> Bus Creator57/1  "Xangularrate"
  4/2(Yangularrate_Out) -> Bus Creator57/2  "Yangularrate"
  5/1(Zangularrate_Out) -> Bus Creator58/1  "Zangularrate"
  5/2(Xacceleration_Out) -> Bus Creator58/2  "Xacceleration"
  6/1(Yacceleration_Out) -> Bus Creator59/1  "Yacceleration"
  6/2(Zacceleration_Out) -> Bus Creator59/2  "Zacceleration"
  7/1(NorthSpd_Out) -> Bus Creator60/1  "NorthSpd"
  7/2(SkySpd_Out) -> Bus Creator60/2  "SkySpd"
  8/1(EastSpd_Out) -> Bus Creator61/1  "EastSpd"
  8/2(Altitude_Out) -> Bus Creator61/2  "Altitude"
  9/1(Longitude_Out) -> Bus Creator62/1  "Longitude"
  9/2(Latitude_Out) -> Bus Creator62/2  "Latitude"
  10/1(Rolling_Out) -> Bus Creator63/1  "Rolling"
  10/2(Heading_Out) -> Bus Creator63/2  "Heading"
  Bus Creator57/1 -> Bus Creator64/1  "IMU1"
  Bus Creator58/1 -> Bus Creator64/2  "IMU2"
  Bus Creator59/1 -> Bus Creator64/3  "IMU3"
  Bus Creator60/1 -> Bus Creator64/4  "IMU4"
  Bus Creator61/1 -> Bus Creator64/5  "IMU5"
  Bus Creator62/1 -> Bus Creator64/6  "IMU6"
  Bus Creator63/1 -> Bus Creator64/7  "IMU7"
  11/1(Pitching_Out) -> Bus Creator65/1  "Pitching"
  Bus Creator65/1 -> Bus Creator64/8  "IMU8"
  Bus Creator64/1 -> Bus Creator44/5  "IMU"

== matlab function six_plus_six_AcmsteeringV09_main_2lfrf/MainControl/mode_control/backward/backward/Drive/左右侧电机分配及功率限制/MATLAB Function ==
  data: trqlim_l input; trq_dem_l output; trq_dem_r output; trq_dem_l1 input; trqlim_r input; trq_dem_r1 input; delta_T_dem input
function [trq_dem_l,trq_dem_r] = fcn(trqlim_l,trq_dem_l1,trqlim_r,trq_dem_r1,delta_T_dem)
%#codegen
if trq_dem_l1==trqlim_l
    trq_dem_l=single(trq_dem_l1);
    trq_dem_r=single(trq_dem_l1+delta_T_dem);%这时候加的是负值
elseif trq_dem_r1==trqlim_r
    trq_dem_l=single(trq_dem_r1-delta_T_dem);
    trq_dem_r=single(trq_dem_r1);
    
else
    trq_dem_l=single(trq_dem_l1);
    trq_dem_r=single(trq_dem_r1);
end
% trq_dem_l=single(max(0,trq_dem_l));%限一下最小值，不要小于0
% trq_dem_r=single(max(0,trq_dem_r));
trq_dem_l=single(max(-trqlim_l,trq_dem_l));%小转向半径下，内侧履带是可能输出负转矩的，从地面吸收功率，给外侧，所以不能限到0，限到最大电机外特性负值
trq_dem_r=single(max(-trqlim_r,trq_dem_r));
end

== matlab function six_plus_six_AcmsteeringV09_main_2lfrf/MainControl/mode_control/backward/backward/Drive/目标转向力矩确定模块/MATLAB Function1 ==
  data: v_act input; Rturn_min_ag output; ag_thr input
 function Rturn_min_ag = fcn(v_act,ag_thr)
%#codegen

    Rturn_min_ag=single((v_act/3.6)^2/ag_thr);
end

== matlab function six_plus_six_AcmsteeringV09_main_2lfrf/MainControl/mode_control/forward/forward/MATLAB Function ==
  data: acc_dem input; y output; brake_dem input; HAC input
function y = fcn(acc_dem,brake_dem,HAC)
%#codegen
if HAC==1
    if acc_dem>0
        y=int8(0);
    else
        y=int8(1);
    end
else
    if brake_dem==0
        y=int8(0);
    else
        y=int8(1);
    end
end
end

== matlab function six_plus_six_AcmsteeringV09_main_2lfrf/MainControl/mode_control/backward/backward/Drive/驱动防滑控制TCS/直行TCS/直行/HeartBeat3 ==
  data: life_pre input; life output
function life = fcn(life_pre)
%#codegen
life=single(life_pre+1);
if life>255
    life=single(0);
end
end

== matlab function six_plus_six_AcmsteeringV09_main_2lfrf/MainControl/mode_control/backward/backward/MATLAB Function ==
  data: acc_dem input; y output; brake_dem input; HAC input
function y = fcn(acc_dem,brake_dem,HAC)
%#codegen
if HAC==1
    if acc_dem<0
        y=int8(0);
    else
        y=int8(1);
    end
else
    if brake_dem==0
        y=int8(0);
    else
        y=int8(1);
    end
end
end

== matlab function six_plus_six_AcmsteeringV09_main_2lfrf/MainControl/mode_control/center_steer/center_steer/HeartBeat ==
  data: life_pre input; life output
function life = fcn(life_pre)
%#codegen
life=single(life_pre+1);
if life>255
    life=single(0);
end
end

== matlab function six_plus_six_AcmsteeringV09_main_2lfrf/MainControl/mode_control/center_steer/center_steer/HeartBeat5 ==
  data: life_pre input; life output
function life = fcn(life_pre)
%#codegen
life=single(life_pre+1);
if life>255
    life=single(0);
end
end

== matlab function six_plus_six_AcmsteeringV09_main_2lfrf/MainControl/mode_control/emergency_stop/emergency_stop/HeartBeat3 ==
  data: life_pre input; life output
function life = fcn(life_pre)
%#codegen
life=single(life_pre+1);
if life>255
    life=single(0);
end
end
